simulink model "sensibility_functions"  (Simulink 6.6)
settings: Solver=ode45  StartTime=0.0  StopTime=12  RelTol=1e-3
settings Model: Creator=mxkana  LastModifiedBy=mxkana

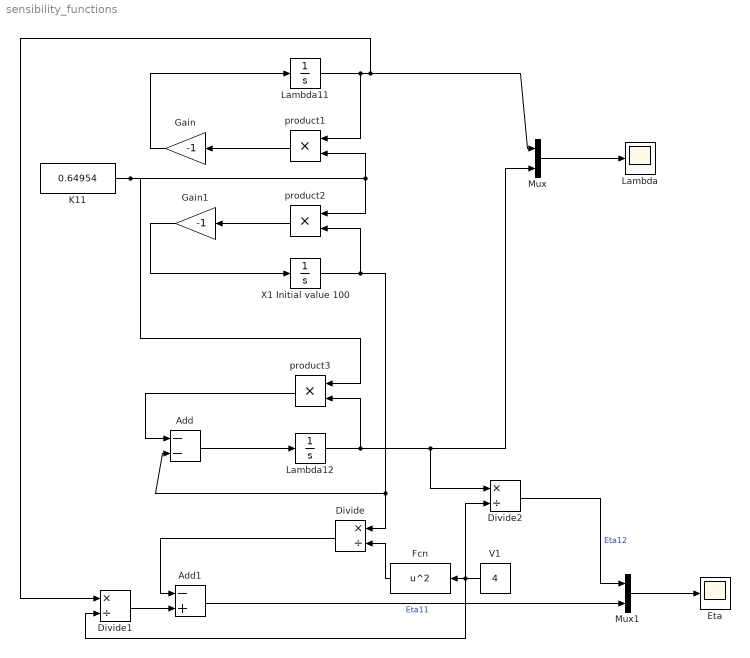
== system sensibility_functions ==
  Add : Sum  Inputs=--  OutScaling=2^-10
  Add1 : Sum  Inputs=-+  OutScaling=2^-10
  Divide : Product  Orientation=left  Inputs=*/  OutScaling=2^-10
  Divide1 : Product  Inputs=*/  OutScaling=2^-10
  Divide2 : Product  Inputs=*/  OutScaling=2^-10
  Eta : Scope
  Fcn : Fcn  Orientation=left  Expr=u^2
  Gain : Gain  Orientation=left  Gain=-1
  Gain1 : Gain  Orientation=left  Gain=-1
  K11 : Constant  Value=0.64954
  Lambda : Scope
  Lambda11 : Integrator
  Lambda12 : Integrator
  Mux : Mux  Inputs=2
  Mux1 : Mux  Inputs=2
  V1 : Constant  Orientation=left  Value=4
  X1 Initial value 100 : Integrator  InitialCondition=100
  product1 : Product  Orientation=left  Inputs=**  OutScaling=2^-10
  product2 : Product  Orientation=left  Inputs=**  OutScaling=2^-10
  product3 : Product  Orientation=left  Inputs=**  OutScaling=2^-10
  wires:
  product1/1 -> Gain/1
  Gain/1 -> Lambda11/1
  Lambda11/1 -> product1/1, Mux/1, Divide1/1
  X1 Initial value 100/1 -> product2/2, Add/2, Divide/1
  K11/1 -> product1/2, product2/1, product3/1
  product2/1 -> Gain1/1
  Lambda12/1 -> product3/2, Mux/2, Divide2/1
  Add/1 -> Lambda12/1
  product3/1 -> Add/1
  Mux/1 -> Lambda/1
  Fcn/1 -> Divide/2
  Divide/1 -> Add1/1
  Add1/1 -> Mux1/2  "Eta11"
  Divide1/1 -> Add1/2
  V1/1 -> Divide2/2, Divide1/2, Fcn/1
  Divide2/1 -> Mux1/1  "Eta12"
  Mux1/1 -> Eta/1
  Gain1/1 -> X1 Initial value 100/1
